simulink model "Radar"  (R2022a)
settings: Solver=VariableStepAuto  StartTime=0.0  StopTime=inf  RelTol=1e-3
libraries: spsSawtoothGeneratorLib x1
settings Model: Creator=fercl  LastModifiedBy=fercl

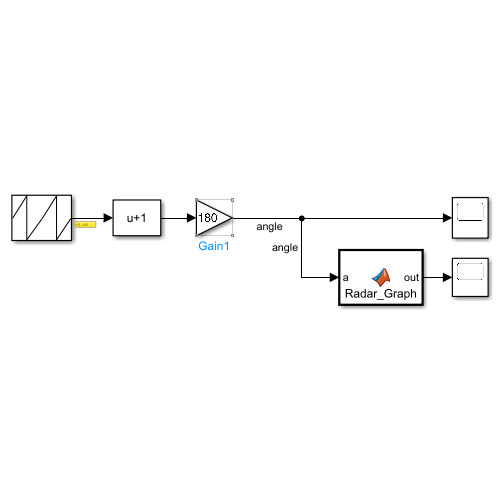
[thumbnail: Simulink's stored preview of the top-level diagram]
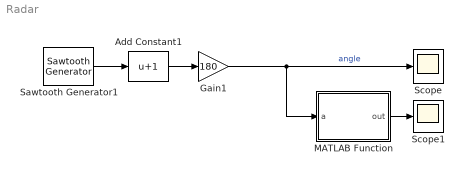
== system Radar ==
  Add Constant1 : Bias  Bias=1  SaturateOnIntegerOverflow=off
  Gain1 : Gain  Gain=180
  MATLAB Function : MATLAB Function  TreatAsAtomicUnit=on  SystemSampleTime=0.1
  Sawtooth Generator1 : spsSawtoothGeneratorLib/Sawtooth Generator  Freq=0.1  Phase=180  Ts=0
  Scope : Scope
  Scope1 : Scope
  wires:
  Gain1/1 -> MATLAB Function/1(a), Scope/1  "angle"
  Sawtooth Generator1/1 -> Add Constant1/1
  Add Constant1/1 -> Gain1/1
  MATLAB Function/1(out) -> Scope1/1

== matlab function Radar/MATLAB Function ==
  data: a input; out output
function out = Radar_Graph(a)
    tic
    xl = 20*cosd(a);
%     x = linspace(0,xl,2);
    yl = 20*sind(a);
%     y = linspace(0,yl,2);
    plot([0 xl], [0 yl])
    xlim([-20 20])
    ylim([-20 20])
    out = toc;
